simulink model "Vehicle_Dynamics_Tests_org"  (Simulink 10.0)
settings: Solver=ode15s  StartTime=0.0  StopTime=10  MaxStep=0.01  RelTol=1e-4  AbsTol=1e-4  EnableMultiTasking=on
PostLoadFcn:
  | Configure_TNO_Tire_Test('handling');
undefined symbols (not defined in the file): angparking, delta, is, TNO_Veh_PARAM, tparking, tswd, tvxset, vxset, X, Y, Z
libraries: sm_lib x54, nesl_utility x25, Delft_Tyre_sm2glib x16
(part 2 of 2)

== system Vehicle_Dynamics_Tests_org/HubRF ==
  Hub : sm_lib/Body Elements/Cylindrical Solid  GraphicAmbientColor=[0.15 0.15 0.15 1.0]  BasedOnType=Density  CenterOfMass=[0 0 0]  CenterOfMassUnits=m  GraphicDiffuseColor=[0.2 0.8 1.0]  CylinderLength=TNO_Veh_PARAM.Hub.Length  CylinderLengthUnits=m  CylinderRadius=TNO_Veh_PARAM.Hub.Radius  CylinderRadiusUnits=m  Density=1000  DensityUnits=kg/(m^3)  DoExposeReferenceFrame=on  GraphicEmissiveColor=[0.0 0.0 0.0 1.0]  ExportEntireGeometry=off  SerializedFrames=<Frames/>  MarkerShape=Sphere  MarkerSize=10  GraphicType=FromGeometry  InertiaType=CalculateFromGeometry  Mass=1  MassUnits=kg  MomentsOfInertia=[1 1 1]  MomentsOfInertiaUnits=kg*m^2  GraphicOpacity=1.0  ProductsOfInertia=[0 0 0]  ProductsOfInertiaUnits=kg*m^2  GraphicShininess=75  GraphicSpecularColor=[0.5 0.5 0.5 1.0]  GraphicVisPropType=SimpleVisualProperties
  Transform (Whl) : sm_lib/Frames and Transforms/Rigid Transform  TranslationMethod=None  TranslationStandardOffset=0  TranslationLengthUnit=m  TranslationStandardAxis=+Z  TranslationCartesianOffset=[0 0 0]  TranslationROffset=0  TranslationROffsetUnits=m  TranslationZOffset=0  TranslationZOffsetUnits=m  TranslationThetaOffset=0  TranslationThetaOffsetUnits=deg  RotationMethod=StandardAxis  RotationAngleUnits=deg  RotationStandardAxis=-X  RotationAngle=90  RotationArbitraryAxis=[0 0 1]  FollAlignAxisA=+X  BaseAlignAxisA=+Y  FollAlignAxisB=+Y  BaseAlignAxisB=+Z  RotationSequenceAxes=FollowerAxes  RotationSequence=XYX  RotationSequenceAngles=[0 0 0]  RotationSequenceAnglesUnits=deg  RotationMatrix=[1 0 0; 0 1 0; 0 0 1]
  Transform1 (Whl) : sm_lib/Frames and Transforms/Rigid Transform  TranslationMethod=None  TranslationStandardOffset=0  TranslationLengthUnit=m  TranslationStandardAxis=+Z  TranslationCartesianOffset=[0 0 0]  TranslationROffset=0  TranslationROffsetUnits=m  TranslationZOffset=0  TranslationZOffsetUnits=m  TranslationThetaOffset=0  TranslationThetaOffsetUnits=deg  RotationMethod=StandardAxis  RotationAngleUnits=deg  RotationStandardAxis=+Z  RotationAngle=180  RotationArbitraryAxis=[0 0 1]  FollAlignAxisA=+X  BaseAlignAxisA=+Y  FollAlignAxisB=+Y  BaseAlignAxisB=+Z  RotationSequenceAxes=FollowerAxes  RotationSequence=XYX  RotationSequenceAngles=[0 0 0]  RotationSequenceAnglesUnits=deg  RotationMatrix=[1 0 0; 0 1 0; 0 0 1]
  Axle : PMIOPort  Side=Left
  Whl : PMIOPort  Port=2  Side=Right
  connections:
  Hub/RConn1 -- Axle/RConn1 -- Transform1 (Whl)/LConn1
  Transform (Whl)/LConn1 -- Transform1 (Whl)/RConn1
  Whl/RConn1 -- Transform (Whl)/RConn1

== system Vehicle_Dynamics_Tests_org/Maneuver selection ==

== system Vehicle_Dynamics_Tests_org/Plot Tire Results ==

== system Vehicle_Dynamics_Tests_org/RA Housing ==
  Axle Ctr : sm_lib/Body Elements/Cylindrical Solid  GraphicAmbientColor=[0.15 0.15 0.15 1.0]  BasedOnType=Density  CenterOfMass=[0 0 0]  CenterOfMassUnits=m  GraphicDiffuseColor=[0.6 0.6 0.6]  CylinderLength=TNO_Veh_PARAM.Axle_Housing.Length  CylinderLengthUnits=m  CylinderRadius=TNO_Veh_PARAM.Axle_Housing.Radius  CylinderRadiusUnits=m  Density=1000  DensityUnits=kg/(m^3)  DoExposeReferenceFrame=on  GraphicEmissiveColor=[0.0 0.0 0.0 1.0]  ExportEntireGeometry=off  SerializedFrames=<Frames/>  MarkerShape=Sphere  MarkerSize=10  GraphicType=FromGeometry  InertiaType=CalculateFromGeometry  Mass=1  MassUnits=kg  MomentsOfInertia=[1 1 1]  MomentsOfInertiaUnits=kg*m^2  GraphicOpacity=1.0  ProductsOfInertia=[0 0 0]  ProductsOfInertiaUnits=kg*m^2  GraphicShininess=75  GraphicSpecularColor=[0.5 0.5 0.5 1.0]  GraphicVisPropType=SimpleVisualProperties
  Transform (Body) : sm_lib/Frames and Transforms/Rigid Transform  TranslationMethod=None  TranslationStandardOffset=0  TranslationLengthUnit=m  TranslationStandardAxis=+Z  TranslationCartesianOffset=[0 0.05 0]  TranslationROffset=0  TranslationROffsetUnits=m  TranslationZOffset=0  TranslationZOffsetUnits=m  TranslationThetaOffset=0  TranslationThetaOffsetUnits=deg  RotationMethod=StandardAxis  RotationAngleUnits=deg  RotationStandardAxis=+X  RotationAngle=90  RotationArbitraryAxis=[0 0 1]  FollAlignAxisA=+X  BaseAlignAxisA=+Y  FollAlignAxisB=+Y  BaseAlignAxisB=+Z  RotationSequenceAxes=FollowerAxes  RotationSequence=XYX  RotationSequenceAngles=[0 0 0]  RotationSequenceAnglesUnits=deg  RotationMatrix=[1 0 0; 0 1 0; 0 0 1]
  Transform (RA) : sm_lib/Frames and Transforms/Rigid Transform  TranslationMethod=StandardAxis  TranslationStandardOffset=TNO_Veh_PARAM.Suspension.RA.Roll.Height  TranslationLengthUnit=m  TranslationStandardAxis=+Y  TranslationCartesianOffset=[0 0.05 0]  TranslationROffset=0  TranslationROffsetUnits=m  TranslationZOffset=0  TranslationZOffsetUnits=m  TranslationThetaOffset=0  TranslationThetaOffsetUnits=deg  RotationMethod=StandardAxis  RotationAngleUnits=deg  RotationStandardAxis=+Y  RotationAngle=90  RotationArbitraryAxis=[0 0 1]  FollAlignAxisA=+X  BaseAlignAxisA=+Y  FollAlignAxisB=+Y  BaseAlignAxisB=+Z  RotationSequenceAxes=FollowerAxes  RotationSequence=XYX  RotationSequenceAngles=[0 0 0]  RotationSequenceAnglesUnits=deg  RotationMatrix=[1 0 0; 0 1 0; 0 0 1]
  Body : PMIOPort  Side=Left
  RA : PMIOPort  Port=2  Side=Right
  connections:
  RA/RConn1 -- Transform (RA)/RConn1
  Transform (Body)/LConn1 -- Axle Ctr/RConn1 -- Transform (RA)/LConn1
  Transform (Body)/RConn1 -- Body/RConn1

== system Vehicle_Dynamics_Tests_org/RHeave ==
  PS-Simulink Converter14 : nesl_utility/PS-Simulink Converter  PhysicalDomain=network_engine_domain  SubClassName=ps_output  LeftPortType=input  RightPortType=output  PseudoPeriodic=off  Frequencies=[]  Unit=m  AffineConversion=off
  To Workspace4 : ToWorkspace  VariableName=RAheave  SampleTime=-1
  Conn1 : PMIOPort  Side=Left
  wires:
  PS-Simulink Converter14/1 -> To Workspace4/1
  connections:
  Conn1/RConn1 -- PS-Simulink Converter14/LConn1

== system Vehicle_Dynamics_Tests_org/RRoll ==
  PS-Simulink Converter16 : nesl_utility/PS-Simulink Converter  PhysicalDomain=network_engine_domain  SubClassName=ps_output  LeftPortType=input  RightPortType=output  PseudoPeriodic=off  Frequencies=[]  Unit=deg  AffineConversion=off
  To Workspace2 : ToWorkspace  VariableName=RAroll  SampleTime=-1
  Conn1 : PMIOPort  Side=Right
  wires:
  PS-Simulink Converter16/1 -> To Workspace2/1
  connections:
  Conn1/RConn1 -- PS-Simulink Converter16/LConn1

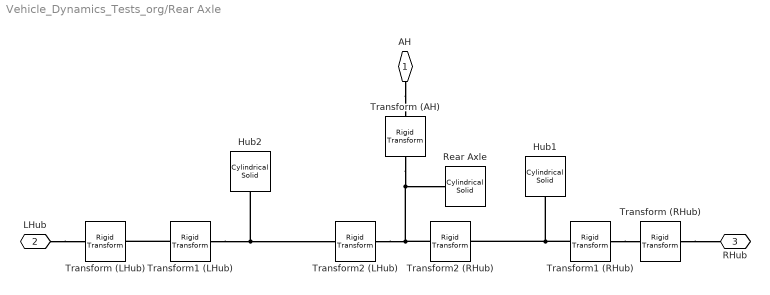
== system Vehicle_Dynamics_Tests_org/Rear Axle ==
  Hub1 : sm_lib/Body Elements/Cylindrical Solid  GraphicAmbientColor=[0.15 0.15 0.15 1.0]  BasedOnType=Density  CenterOfMass=[0 0 0]  CenterOfMassUnits=m  GraphicDiffuseColor=[0.2 0.8 1.0]  CylinderLength=TNO_Veh_PARAM.Hub.Length  CylinderLengthUnits=m  CylinderRadius=TNO_Veh_PARAM.Hub.Radius  CylinderRadiusUnits=m  Density=1000  DensityUnits=kg/(m^3)  DoExposeReferenceFrame=on  GraphicEmissiveColor=[0.0 0.0 0.0 1.0]  ExportEntireGeometry=off  SerializedFrames=<Frames/>  MarkerShape=Sphere  MarkerSize=10  GraphicType=FromGeometry  InertiaType=CalculateFromGeometry  Mass=1  MassUnits=kg  MomentsOfInertia=[1 1 1]  MomentsOfInertiaUnits=kg*m^2  GraphicOpacity=1.0  ProductsOfInertia=[0 0 0]  ProductsOfInertiaUnits=kg*m^2  GraphicShininess=75  GraphicSpecularColor=[0.5 0.5 0.5 1.0]  GraphicVisPropType=SimpleVisualProperties
  Hub2 : sm_lib/Body Elements/Cylindrical Solid  GraphicAmbientColor=[0.15 0.15 0.15 1.0]  BasedOnType=Density  CenterOfMass=[0 0 0]  CenterOfMassUnits=m  GraphicDiffuseColor=[0.2 0.8 1.0]  CylinderLength=TNO_Veh_PARAM.Hub.Length  CylinderLengthUnits=m  CylinderRadius=TNO_Veh_PARAM.Hub.Radius  CylinderRadiusUnits=m  Density=1000  DensityUnits=kg/(m^3)  DoExposeReferenceFrame=on  GraphicEmissiveColor=[0.0 0.0 0.0 1.0]  ExportEntireGeometry=off  SerializedFrames=<Frames/>  MarkerShape=Sphere  MarkerSize=10  GraphicType=FromGeometry  InertiaType=CalculateFromGeometry  Mass=1  MassUnits=kg  MomentsOfInertia=[1 1 1]  MomentsOfInertiaUnits=kg*m^2  GraphicOpacity=1.0  ProductsOfInertia=[0 0 0]  ProductsOfInertiaUnits=kg*m^2  GraphicShininess=75  GraphicSpecularColor=[0.5 0.5 0.5 1.0]  GraphicVisPropType=SimpleVisualProperties
  Rear Axle : sm_lib/Body Elements/Cylindrical Solid  GraphicAmbientColor=[0.15 0.15 0.15 1.0]  BasedOnType=Density  CenterOfMass=[0 0 0]  CenterOfMassUnits=m  GraphicDiffuseColor=[0.6 0.6 0.6]  CylinderLength=TNO_Veh_PARAM.Axle.RA.Length  CylinderLengthUnits=m  CylinderRadius=TNO_Veh_PARAM.Axle.RA.Radius  CylinderRadiusUnits=m  Density=1000  DensityUnits=kg/(m^3)  DoExposeReferenceFrame=on  GraphicEmissiveColor=[0.0 0.0 0.0 1.0]  ExportEntireGeometry=off  SerializedFrames=<Frames/>  MarkerShape=Sphere  MarkerSize=10  GraphicType=FromGeometry  InertiaType=Custom  Mass=TNO_Veh_PARAM.Axle.RA.Mass  MassUnits=kg  MomentsOfInertia=TNO_Veh_PARAM.Axle.RA.Inertia  MomentsOfInertiaUnits=kg*m^2  GraphicOpacity=1.0  ProductsOfInertia=[0 0 0]  ProductsOfInertiaUnits=kg*m^2  GraphicShininess=75  GraphicSpecularColor=[0.5 0.5 0.5 1.0]  GraphicVisPropType=SimpleVisualProperties
  Transform (AH) : sm_lib/Frames and Transforms/Rigid Transform  TranslationMethod=StandardAxis  TranslationStandardOffset=TNO_Veh_PARAM.Axle.RA.Height  TranslationLengthUnit=m  TranslationStandardAxis=+Y  TranslationCartesianOffset=[0 0.225 0]  TranslationROffset=0  TranslationROffsetUnits=m  TranslationZOffset=0  TranslationZOffsetUnits=m  TranslationThetaOffset=0  TranslationThetaOffsetUnits=deg  RotationMethod=StandardAxis  RotationAngleUnits=deg  RotationStandardAxis=+Y  RotationAngle=-90  RotationArbitraryAxis=[0 0 1]  FollAlignAxisA=+X  BaseAlignAxisA=+Y  FollAlignAxisB=+Y  BaseAlignAxisB=+Z  RotationSequenceAxes=FollowerAxes  RotationSequence=XYX  RotationSequenceAngles=[0 0 0]  RotationSequenceAnglesUnits=deg  RotationMatrix=[1 0 0; 0 1 0; 0 0 1]
  Transform (LHub) : sm_lib/Frames and Transforms/Rigid Transform  TranslationMethod=None  TranslationStandardOffset=0  TranslationLengthUnit=m  TranslationStandardAxis=+Z  TranslationCartesianOffset=[0 0 0]  TranslationROffset=0  TranslationROffsetUnits=m  TranslationZOffset=0  TranslationZOffsetUnits=m  TranslationThetaOffset=0  TranslationThetaOffsetUnits=deg  RotationMethod=StandardAxis  RotationAngleUnits=deg  RotationStandardAxis=-X  RotationAngle=90  RotationArbitraryAxis=[0 0 1]  FollAlignAxisA=+X  BaseAlignAxisA=+Y  FollAlignAxisB=+Y  BaseAlignAxisB=+Z  RotationSequenceAxes=FollowerAxes  RotationSequence=XYX  RotationSequenceAngles=[0 0 0]  RotationSequenceAnglesUnits=deg  RotationMatrix=[1 0 0; 0 1 0; 0 0 1]
  Transform (RHub) : sm_lib/Frames and Transforms/Rigid Transform  TranslationMethod=None  TranslationStandardOffset=0  TranslationLengthUnit=m  TranslationStandardAxis=+Z  TranslationCartesianOffset=[0 0 0]  TranslationROffset=0  TranslationROffsetUnits=m  TranslationZOffset=0  TranslationZOffsetUnits=m  TranslationThetaOffset=0  TranslationThetaOffsetUnits=deg  RotationMethod=StandardAxis  RotationAngleUnits=deg  RotationStandardAxis=-X  RotationAngle=90  RotationArbitraryAxis=[0 0 1]  FollAlignAxisA=+X  BaseAlignAxisA=+Y  FollAlignAxisB=+Y  BaseAlignAxisB=+Z  RotationSequenceAxes=FollowerAxes  RotationSequence=XYX  RotationSequenceAngles=[0 0 0]  RotationSequenceAnglesUnits=deg  RotationMatrix=[1 0 0; 0 1 0; 0 0 1]
  Transform1 (LHub) : sm_lib/Frames and Transforms/Rigid Transform  TranslationMethod=None  TranslationStandardOffset=0  TranslationLengthUnit=m  TranslationStandardAxis=+Z  TranslationCartesianOffset=[0 0 0]  TranslationROffset=0  TranslationROffsetUnits=m  TranslationZOffset=0  TranslationZOffsetUnits=m  TranslationThetaOffset=0  TranslationThetaOffsetUnits=deg  RotationMethod=StandardAxis  RotationAngleUnits=deg  RotationStandardAxis=+Z  RotationAngle=180  RotationArbitraryAxis=[0 0 1]  FollAlignAxisA=+X  BaseAlignAxisA=+Y  FollAlignAxisB=+Y  BaseAlignAxisB=+Z  RotationSequenceAxes=FollowerAxes  RotationSequence=XYX  RotationSequenceAngles=[0 0 0]  RotationSequenceAnglesUnits=deg  RotationMatrix=[1 0 0; 0 1 0; 0 0 1]
  Transform1 (RHub) : sm_lib/Frames and Transforms/Rigid Transform  TranslationMethod=None  TranslationStandardOffset=0  TranslationLengthUnit=m  TranslationStandardAxis=+Z  TranslationCartesianOffset=[0 0 0]  TranslationROffset=0  TranslationROffsetUnits=m  TranslationZOffset=0  TranslationZOffsetUnits=m  TranslationThetaOffset=0  TranslationThetaOffsetUnits=deg  RotationMethod=StandardAxis  RotationAngleUnits=deg  RotationStandardAxis=+Z  RotationAngle=180  RotationArbitraryAxis=[0 0 1]  FollAlignAxisA=+X  BaseAlignAxisA=+Y  FollAlignAxisB=+Y  BaseAlignAxisB=+Z  RotationSequenceAxes=FollowerAxes  RotationSequence=XYX  RotationSequenceAngles=[0 0 0]  RotationSequenceAnglesUnits=deg  RotationMatrix=[1 0 0; 0 1 0; 0 0 1]
  Transform2 (LHub) : sm_lib/Frames and Transforms/Rigid Transform  TranslationMethod=StandardAxis  TranslationStandardOffset=-TNO_Veh_PARAM.WheelBase/2  TranslationLengthUnit=m  TranslationStandardAxis=+Z  TranslationCartesianOffset=[0 0 0]  TranslationROffset=0  TranslationROffsetUnits=m  TranslationZOffset=0  TranslationZOffsetUnits=m  TranslationThetaOffset=0  TranslationThetaOffsetUnits=deg  RotationMethod=StandardAxis  RotationAngleUnits=deg  RotationStandardAxis=+X  RotationAngle=90  RotationArbitraryAxis=[0 0 1]  FollAlignAxisA=+X  BaseAlignAxisA=+Y  FollAlignAxisB=+Y  BaseAlignAxisB=+Z  RotationSequenceAxes=FollowerAxes  RotationSequence=XYX  RotationSequenceAngles=[0 0 0]  RotationSequenceAnglesUnits=deg  RotationMatrix=[1 0 0; 0 1 0; 0 0 1]
  Transform2 (RHub) : sm_lib/Frames and Transforms/Rigid Transform  TranslationMethod=StandardAxis  TranslationStandardOffset=TNO_Veh_PARAM.WheelBase/2  TranslationLengthUnit=m  TranslationStandardAxis=+Z  TranslationCartesianOffset=[0 0 0]  TranslationROffset=0  TranslationROffsetUnits=m  TranslationZOffset=0  TranslationZOffsetUnits=m  TranslationThetaOffset=0  TranslationThetaOffsetUnits=deg  RotationMethod=StandardAxis  RotationAngleUnits=deg  RotationStandardAxis=+X  RotationAngle=90  RotationArbitraryAxis=[0 0 1]  FollAlignAxisA=+X  BaseAlignAxisA=+Y  FollAlignAxisB=+Y  BaseAlignAxisB=+Z  RotationSequenceAxes=FollowerAxes  RotationSequence=XYX  RotationSequenceAngles=[0 0 0]  RotationSequenceAnglesUnits=deg  RotationMatrix=[1 0 0; 0 1 0; 0 0 1]
  AH : PMIOPort  Side=Left
  LHub : PMIOPort  Port=2  Side=Right
  RHub : PMIOPort  Port=3  Side=Right
  connections:
  AH/RConn1 -- Transform (AH)/RConn1
  Transform2 (LHub)/LConn1 -- Transform (AH)/LConn1 -- Rear Axle/RConn1 -- Transform2 (RHub)/LConn1
  Transform1 (RHub)/LConn1 -- Transform2 (RHub)/RConn1 -- Hub1/RConn1
  Transform1 (LHub)/LConn1 -- Transform2 (LHub)/RConn1 -- Hub2/RConn1
  Transform1 (RHub)/RConn1 -- Transform (RHub)/LConn1
  Transform (RHub)/RConn1 -- RHub/RConn1
  Transform1 (LHub)/RConn1 -- Transform (LHub)/LConn1
  LHub/RConn1 -- Transform (LHub)/RConn1

== system Vehicle_Dynamics_Tests_org/Sensing ==
  Mux : Mux
  Fz : Outport
  wires:
  [RR_Fz] -> Mux/4
  Mux/1 -> Fz/1
  [LF_Fz] -> Mux/1
  [RF_Fz] -> Mux/2
  [LR_Fz] -> Mux/3

== system Vehicle_Dynamics_Tests_org/Steering Input ==
  note: 1) Only subsystems can be added as variant choices at this level
      | 2) Blocks cannot be connected at this level as connectivity is
      | automatically determined at simulation, based on the active variant
  No Steer : Subsystem  VariantControl=NoSteer
  Parking : Subsystem  VariantControl=Parking
  Sine With Dwell : Subsystem  VariantControl=SineWithDwell
  Slalom : Subsystem  VariantControl=Slalom
  Step Steer : Subsystem  VariantControl=StepSteer
  L : PMIOPort  Side=Right
  R : PMIOPort  Port=2  Side=Right

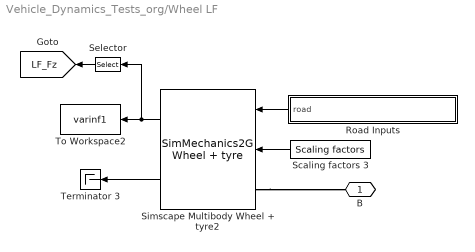
== system Vehicle_Dynamics_Tests_org/Wheel LF ==
  Road Inputs : Subsystem  VariantControlMode=Label  Variant=on  LabelModeActiveChoice=NonMoving
  Scaling factors 3 : Delft_Tyre_sm2glib/SimMechanics 2G/Scaling factors  LMUX=1  LKX=1  LMUY=1  LKY=1  LKYC=1  LTR=1  LKZC=1
  Selector : Selector  InputPortWidth=40  IndexOptions=Index vector (dialog)  Indices=[3]  OutputSizes=1
  Simscape Multibody Wheel + tyre2 : Delft_Tyre_sm2glib/SimMechanics 2G/SimMechanics2G Wheel + tyre  Tag=SimMechanics Wheel + tyre  idtyre=1  inertia=[10 1 2]  tpfname=which('TNO_car205_60R15.tir')  rdfname=which('TNO_FlatRoad.rdf')  side_mode=(1xxx) left  cnt_mode=(x1xx) smooth road  dyn_mode=(xx2x) relaxation behaviour - non-linear  mf_mode=(xxx4) combined  use_mode=1e8  disp_debug=off
  Terminator 3 : Terminator
  To Workspace2 : ToWorkspace  VariableName=varinf1  SampleTime=-1
  B : PMIOPort  Side=Right
  tag scope: LF_Fz=global
  wires:
  Scaling factors 3/1 -> Simscape Multibody Wheel + tyre2/2
  Road Inputs/1(road) -> Simscape Multibody Wheel + tyre2/1
  Simscape Multibody Wheel + tyre2/1 -> Selector/1, To Workspace2/1
  Simscape Multibody Wheel + tyre2/2 -> Terminator 3/1
  Selector/1 -> [LF_Fz]
  connections:
  Simscape Multibody Wheel + tyre2/LConn1 -- B/RConn1

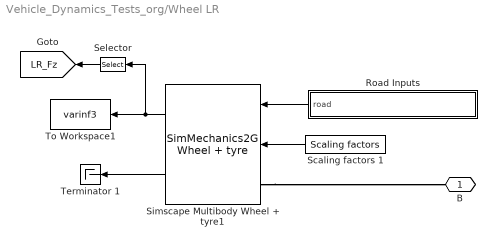
== system Vehicle_Dynamics_Tests_org/Wheel LR ==
  Road Inputs : Subsystem  VariantControlMode=Label  Variant=on  LabelModeActiveChoice=NonMoving
  Scaling factors 1 : Delft_Tyre_sm2glib/SimMechanics 2G/Scaling factors  LMUX=1  LKX=1  LMUY=1  LKY=1  LKYC=1  LTR=1  LKZC=1
  Selector : Selector  InputPortWidth=40  IndexOptions=Index vector (dialog)  Indices=[3]  OutputSizes=1
  Simscape Multibody Wheel + tyre1 : Delft_Tyre_sm2glib/SimMechanics 2G/SimMechanics2G Wheel + tyre  Tag=SimMechanics Wheel + tyre  idtyre=3  inertia=[10 1 2]  tpfname=which('TNO_car205_60R15.tir')  rdfname=which('TNO_FlatRoad.rdf')  side_mode=(1xxx) left  cnt_mode=(x1xx) smooth road  dyn_mode=(xx2x) relaxation behaviour - non-linear  mf_mode=(xxx4) combined  use_mode=1e8  disp_debug=off
  Terminator 1 : Terminator
  To Workspace1 : ToWorkspace  VariableName=varinf3  SampleTime=-1
  B : PMIOPort  Side=Right
  tag scope: LR_Fz=global
  wires:
  Scaling factors 1/1 -> Simscape Multibody Wheel + tyre1/2
  Road Inputs/1(road) -> Simscape Multibody Wheel + tyre1/1
  Simscape Multibody Wheel + tyre1/1 -> Selector/1, To Workspace1/1
  Simscape Multibody Wheel + tyre1/2 -> Terminator 1/1
  Selector/1 -> [LR_Fz]
  connections:
  Simscape Multibody Wheel + tyre1/LConn1 -- B/RConn1

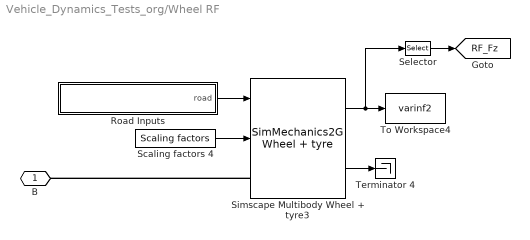
== system Vehicle_Dynamics_Tests_org/Wheel RF ==
  Road Inputs : Subsystem  VariantControlMode=Label  Variant=on  LabelModeActiveChoice=NonMoving
  Scaling factors 4 : Delft_Tyre_sm2glib/SimMechanics 2G/Scaling factors  LMUX=1  LKX=1  LMUY=1  LKY=1  LKYC=1  LTR=1  LKZC=1
  Selector : Selector  InputPortWidth=40  IndexOptions=Index vector (dialog)  Indices=[3]  OutputSizes=1
  Simscape Multibody Wheel + tyre3 : Delft_Tyre_sm2glib/SimMechanics 2G/SimMechanics2G Wheel + tyre  Tag=SimMechanics Wheel + tyre  idtyre=2  inertia=[10 1 2]  tpfname=which('TNO_car205_60R15.tir')  rdfname=which('TNO_FlatRoad.rdf')  side_mode=(2xxx) right  cnt_mode=(x1xx) smooth road  dyn_mode=(xx2x) relaxation behaviour - non-linear  mf_mode=(xxx4) combined  use_mode=1e8  disp_debug=off
  Terminator 4 : Terminator
  To Workspace4 : ToWorkspace  VariableName=varinf2  SampleTime=-1
  B : PMIOPort  Side=Left
  tag scope: RF_Fz=global
  wires:
  Scaling factors 4/1 -> Simscape Multibody Wheel + tyre3/2
  Road Inputs/1(road) -> Simscape Multibody Wheel + tyre3/1
  Simscape Multibody Wheel + tyre3/1 -> Selector/1, To Workspace4/1
  Simscape Multibody Wheel + tyre3/2 -> Terminator 4/1
  Selector/1 -> [RF_Fz]
  connections:
  Simscape Multibody Wheel + tyre3/LConn1 -- B/RConn1

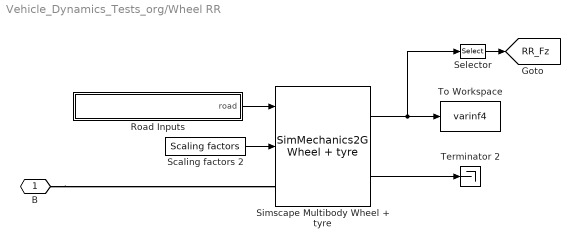
== system Vehicle_Dynamics_Tests_org/Wheel RR ==
  Road Inputs : Subsystem  VariantControlMode=Label  Variant=on  LabelModeActiveChoice=NonMoving
  Scaling factors 2 : Delft_Tyre_sm2glib/SimMechanics 2G/Scaling factors  LMUX=1  LKX=1  LMUY=1  LKY=1  LKYC=1  LTR=1  LKZC=1
  Selector : Selector  InputPortWidth=40  IndexOptions=Index vector (dialog)  Indices=[3]  OutputSizes=1
  Simscape Multibody Wheel + tyre : Delft_Tyre_sm2glib/SimMechanics 2G/SimMechanics2G Wheel + tyre  Tag=SimMechanics Wheel + tyre  idtyre=4  inertia=[10 1 2]  tpfname=which('TNO_car205_60R15.tir')  rdfname=which('TNO_FlatRoad.rdf')  side_mode=(2xxx) right  cnt_mode=(x1xx) smooth road  dyn_mode=(xx2x) relaxation behaviour - non-linear  mf_mode=(xxx4) combined  use_mode=1e8  disp_debug=off
  Terminator 2 : Terminator
  To Workspace : ToWorkspace  VariableName=varinf4  SampleTime=-1
  B : PMIOPort  Side=Left
  tag scope: RR_Fz=global
  wires:
  Scaling factors 2/1 -> Simscape Multibody Wheel + tyre/2
  Road Inputs/1(road) -> Simscape Multibody Wheel + tyre/1
  Simscape Multibody Wheel + tyre/2 -> Terminator 2/1
  Simscape Multibody Wheel + tyre/1 -> Selector/1, To Workspace/1
  Selector/1 -> [RR_Fz]
  connections:
  B/RConn1 -- Simscape Multibody Wheel + tyre/LConn1

== system Vehicle_Dynamics_Tests_org/World ==
  Mechanism Configuration : sm_lib/Utilities/Mechanism Configuration  UniformGravity=Constant  GravityVector=[0 0 -10]  GravityUnits=m/s^2  LinearizationDelta=0.001
  Road : Subsystem  VariantControlMode=Label  Variant=on  LabelModeActiveChoice=NoRoad
  Solver Configuration : nesl_utility/Solver Configuration  PhysicalDomain=network_engine_domain  SubClassName=solver  LeftPortType=input  RightPortType=generic  Tones=[]  Harmonics=[]  SimulateNoise=off  Profile=off  UseLocalSampling=off  EnableSwitchedLinearOptims=on  FrequencyDomain=off  UseCCode=off  RelTol=0.001  AbsTol=1e-06  MinStep=1e-09  ToWorkspace=off  RevertToSquareIcSolve=off  NumHomotopyIterations=100  PhasorMode=off  PhasorModeNumHarmonics=1  DoDC=off  ResidualTolerance=1e-9  UseLocalSolver=off  LocalSolverChoice=NE_BACKWARD_EULER_ADVANCER  LocalSolverSampleTime=.001  DoFixedCost=off  MaxNonlinIter=3  MaxModeIter=2  LinearAlgebra=Sparse  EquationFormulation=NE_TIME_EF  DelaysMemoryBudget=1024  AutomaticFiltering=on  FilteringTimeConstant=0.001  PartitionStorageMethod=AS_NEEDED  PartitionMemoryBudget=1024  PartitionMethod=FAST
  Transform (F) : sm_lib/Frames and Transforms/Rigid Transform  TranslationMethod=Cartesian  TranslationStandardOffset=0.55  TranslationLengthUnit=m  TranslationStandardAxis=+Z  TranslationCartesianOffset=[-TNO_Veh_PARAM.Body.Length/2 0 TNO_Veh_PARAM.Body.Height]  TranslationROffset=0  TranslationROffsetUnits=m  TranslationZOffset=0  TranslationZOffsetUnits=m  TranslationThetaOffset=0  TranslationThetaOffsetUnits=deg  RotationMethod=None  RotationAngleUnits=deg  RotationStandardAxis=+Y  RotationAngle=0  RotationArbitraryAxis=[0 0 1]  FollAlignAxisA=+X  BaseAlignAxisA=+Y  FollAlignAxisB=+Y  BaseAlignAxisB=+Z  RotationSequenceAxes=FollowerAxes  RotationSequence=XYX  RotationSequenceAngles=[0 0 0]  RotationSequenceAnglesUnits=deg  RotationMatrix=[1 0 0; 0 1 0; 0 0 1]
  World Frame : sm_lib/Frames and Transforms/World Frame
  F : PMIOPort  Side=Left
  connections:
  Transform (F)/RConn1 -- F/RConn1
  World Frame/RConn1 -- Road/RConn1 -- Transform (F)/LConn1 -- Solver Configuration/RConn1 -- Mechanism Configuration/RConn1

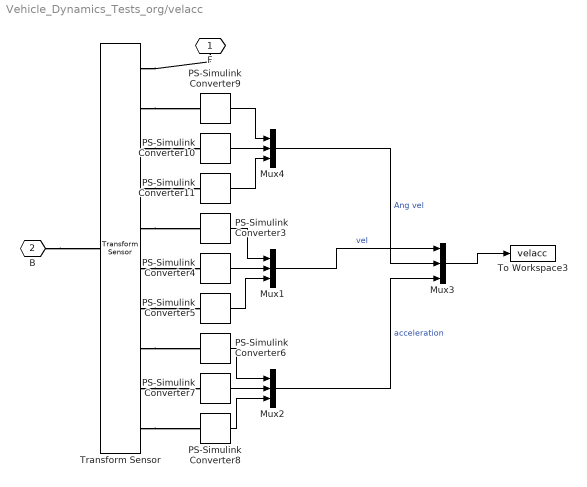
== system Vehicle_Dynamics_Tests_org/velacc ==
  Mux{1..4} (4 alike) : Mux  Inputs=3
  PS-Simulink Converter10 : nesl_utility/PS-Simulink Converter  PhysicalDomain=network_engine_domain  SubClassName=ps_output  LeftPortType=input  RightPortType=output  PseudoPeriodic=off  Frequencies=[]  Unit=deg/s  AffineConversion=off
  PS-Simulink Converter11 : nesl_utility/PS-Simulink Converter  PhysicalDomain=network_engine_domain  SubClassName=ps_output  LeftPortType=input  RightPortType=output  PseudoPeriodic=off  Frequencies=[]  Unit=deg/s  AffineConversion=off
  PS-Simulink Converter3 : nesl_utility/PS-Simulink Converter  PhysicalDomain=network_engine_domain  SubClassName=ps_output  LeftPortType=input  RightPortType=output  PseudoPeriodic=off  Frequencies=[]  Unit=m/s  AffineConversion=off
  PS-Simulink Converter4 : nesl_utility/PS-Simulink Converter  PhysicalDomain=network_engine_domain  SubClassName=ps_output  LeftPortType=input  RightPortType=output  PseudoPeriodic=off  Frequencies=[]  Unit=m/s  AffineConversion=off
  PS-Simulink Converter5 : nesl_utility/PS-Simulink Converter  PhysicalDomain=network_engine_domain  SubClassName=ps_output  LeftPortType=input  RightPortType=output  PseudoPeriodic=off  Frequencies=[]  Unit=m/s  AffineConversion=off
  PS-Simulink Converter6 : nesl_utility/PS-Simulink Converter  PhysicalDomain=network_engine_domain  SubClassName=ps_output  LeftPortType=input  RightPortType=output  PseudoPeriodic=off  Frequencies=[]  Unit=m/s^2  AffineConversion=off
  PS-Simulink Converter7 : nesl_utility/PS-Simulink Converter  PhysicalDomain=network_engine_domain  SubClassName=ps_output  LeftPortType=input  RightPortType=output  PseudoPeriodic=off  Frequencies=[]  Unit=m/s^2  AffineConversion=off
  PS-Simulink Converter8 : nesl_utility/PS-Simulink Converter  PhysicalDomain=network_engine_domain  SubClassName=ps_output  LeftPortType=input  RightPortType=output  PseudoPeriodic=off  Frequencies=[]  Unit=m/s^2  AffineConversion=off
  PS-Simulink Converter9 : nesl_utility/PS-Simulink Converter  PhysicalDomain=network_engine_domain  SubClassName=ps_output  LeftPortType=input  RightPortType=output  PseudoPeriodic=off  Frequencies=[]  Unit=deg/s  AffineConversion=off
  To Workspace3 : ToWorkspace  VariableName=velacc  SampleTime=-1
  Transform Sensor : sm_lib/Frames and Transforms/Transform Sensor  MeasurementFrame=NonRotatingFollower  SenseAngle=off  SenseAxis=off  SenseAngle1=off  SenseAngle2=off  SenseAngle3=off  SenseQ=off  SenseR=off  SenseOmegaX=on  SenseOmegaY=on  SenseOmegaZ=on  SenseOmega1=off  SenseOmega2=off  SenseOmega3=off  SenseQDot=off  SenseRDot=off  SenseAlphaX=off  SenseAlphaY=off  SenseAlphaZ=off  SenseAlpha1=off  SenseAlpha2=off  SenseAlpha3=off  SenseQDDot=off  SenseRDDot=off  SenseX=off  SenseY=off  SenseZ=off  SenseRad=off  SenseAzim=off  SenseDist=off  SenseInc=off  SenseXDot=on  SenseYDot=on  SenseZDot=on  SenseRadDot=off  SenseAzimDot=off  SenseDistDot=off  SenseIncDot=off  SenseXDDot=on  SenseYDDot=on  SenseZDDot=on  SenseRadDDot=off  SenseAzimDDot=off  SenseDistDDot=off  SenseIncDDot=off
  F : PMIOPort  Side=Right
  B : PMIOPort  Port=2  Side=Left
  wires:
  PS-Simulink Converter5/1 -> Mux1/3
  PS-Simulink Converter6/1 -> Mux2/1
  Mux4/1 -> Mux3/2  "Ang vel"
  Mux1/1 -> Mux3/1  "vel"
  Mux2/1 -> Mux3/3  "acceleration"
  Mux3/1 -> To Workspace3/1
  PS-Simulink Converter7/1 -> Mux2/2
  PS-Simulink Converter4/1 -> Mux1/2
  PS-Simulink Converter3/1 -> Mux1/1
  PS-Simulink Converter8/1 -> Mux2/3
  PS-Simulink Converter11/1 -> Mux4/3
  PS-Simulink Converter9/1 -> Mux4/1
  PS-Simulink Converter10/1 -> Mux4/2
  connections:
  Transform Sensor/RConn9 -- PS-Simulink Converter7/LConn1
  Transform Sensor/RConn8 -- PS-Simulink Converter6/LConn1
  Transform Sensor/RConn5 -- PS-Simulink Converter3/LConn1
  Transform Sensor/RConn7 -- PS-Simulink Converter5/LConn1
  Transform Sensor/RConn6 -- PS-Simulink Converter4/LConn1
  Transform Sensor/RConn10 -- PS-Simulink Converter8/LConn1
  B/RConn1 -- Transform Sensor/LConn1
  Transform Sensor/RConn1 -- F/RConn1
  Transform Sensor/RConn2 -- PS-Simulink Converter9/LConn1
  Transform Sensor/RConn3 -- PS-Simulink Converter10/LConn1
  Transform Sensor/RConn4 -- PS-Simulink Converter11/LConn1

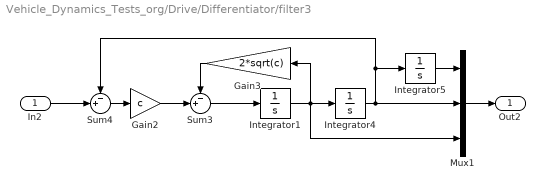
== system Vehicle_Dynamics_Tests_org/Drive/Differentiator/filter3 ==
  In2 : Inport
  Gain2 : Gain  Gain=c  SaturateOnIntegerOverflow=on  OutDataTypeStr=Inherit: Same as input  ParamDataTypeStr=Inherit: Same as input
  Gain3 : Gain  Gain=2*sqrt(c)  SaturateOnIntegerOverflow=on  OutDataTypeStr=Inherit: Same as input  ParamDataTypeStr=Inherit: Same as input
  Integrator1 : Integrator
  Integrator4 : Integrator
  Integrator5 : Integrator  InitialCondition=-1.5
  Mux1 : Mux  Inputs=3
  Sum3 : Sum  Inputs=-+|  SaturateOnIntegerOverflow=on
  Sum4 : Sum  Inputs=-+|  SaturateOnIntegerOverflow=on
  Out2 : Outport
  wires:
  Integrator5/1 -> Mux1/1
  Gain2/1 -> Sum3/2
  Gain3/1 -> Sum3/1
  In2/1 -> Sum4/2
  Sum4/1 -> Gain2/1
  Sum3/1 -> Integrator1/1
  Mux1/1 -> Out2/1
  Integrator4/1 -> Integrator5/1, Sum4/1, Mux1/2
  Integrator1/1 -> Mux1/3, Integrator4/1, Gain3/1

== system Vehicle_Dynamics_Tests_org/Steering Input/No Steer ==
  Constant : Constant  Value=0
  Constant1 : Constant  Value=0
  Simulink-PS Converter : nesl_utility/Simulink-PS Converter  PhysicalDomain=network_engine_domain  SubClassName=ps_input  LeftPortType=input  RightPortType=output  PseudoPeriodic=off  Frequencies=[]  NoiseDistribution=none  NoiseParameters=[]  Unit=rad  AffineConversion=off  FilteringAndDerivatives=filter  SimscapeFilterOrder=2  InputFilterTimeConstant=0.0055  UdotUserProvided=2
  Simulink-PS Converter1 : nesl_utility/Simulink-PS Converter  PhysicalDomain=network_engine_domain  SubClassName=ps_input  LeftPortType=input  RightPortType=output  PseudoPeriodic=off  Frequencies=[]  NoiseDistribution=none  NoiseParameters=[]  Unit=rad  AffineConversion=off  FilteringAndDerivatives=filter  SimscapeFilterOrder=2  InputFilterTimeConstant=0.0055  UdotUserProvided=2
  L : PMIOPort  Side=Right
  R : PMIOPort  Port=2  Side=Right
  wires:
  Constant1/1 -> Simulink-PS Converter/1
  Constant/1 -> Simulink-PS Converter1/1
  connections:
  Simulink-PS Converter1/RConn1 -- L/RConn1
  Simulink-PS Converter/RConn1 -- R/RConn1

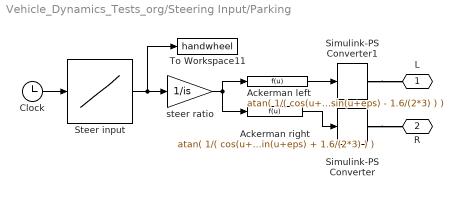
== system Vehicle_Dynamics_Tests_org/Steering Input/Parking ==
  Ackerman left : Fcn  Expr=atan( 1/( cos(u+eps)/sin(u+eps) - 1.6/(2*3) ) )
  Ackerman right : Fcn  Expr=atan( 1/( cos(u+eps)/sin(u+eps) + 1.6/(2*3) ) )
  Clock : Clock
  Simulink-PS Converter : nesl_utility/Simulink-PS Converter  PhysicalDomain=network_engine_domain  SubClassName=ps_input  LeftPortType=input  RightPortType=output  PseudoPeriodic=off  Frequencies=[]  NoiseDistribution=none  NoiseParameters=[]  Unit=rad  AffineConversion=off  FilteringAndDerivatives=filter  SimscapeFilterOrder=2  InputFilterTimeConstant=0.0055  UdotUserProvided=2
  Simulink-PS Converter1 : nesl_utility/Simulink-PS Converter  PhysicalDomain=network_engine_domain  SubClassName=ps_input  LeftPortType=input  RightPortType=output  PseudoPeriodic=off  Frequencies=[]  NoiseDistribution=none  NoiseParameters=[]  Unit=rad  AffineConversion=off  FilteringAndDerivatives=filter  SimscapeFilterOrder=2  InputFilterTimeConstant=0.0055  UdotUserProvided=2
  Steer input : Lookup  InputValues=tparking  Table=angparking
  To Workspace11 : ToWorkspace  VariableName=handwheel  SampleTime=-1
  steer ratio : Gain  Gain=1/is
  L : PMIOPort  Side=Right
  R : PMIOPort  Port=2  Side=Right
  wires:
  Clock/1 -> Steer input/1
  Steer input/1 -> steer ratio/1, To Workspace11/1
  steer ratio/1 -> Ackerman left/1, Ackerman right/1
  Ackerman left/1 -> Simulink-PS Converter1/1
  Ackerman right/1 -> Simulink-PS Converter/1
  connections:
  Simulink-PS Converter/RConn1 -- R/RConn1
  Simulink-PS Converter1/RConn1 -- L/RConn1

== system Vehicle_Dynamics_Tests_org/Steering Input/Sine With Dwell ==
  Clock : Clock
  Simulink-PS Converter : nesl_utility/Simulink-PS Converter  PhysicalDomain=network_engine_domain  SubClassName=ps_input  LeftPortType=input  RightPortType=output  PseudoPeriodic=off  Frequencies=[]  NoiseDistribution=none  NoiseParameters=[]  Unit=rad  AffineConversion=off  FilteringAndDerivatives=filter  SimscapeFilterOrder=2  InputFilterTimeConstant=0.0055  UdotUserProvided=2
  Sine with Dwell Steer input : Lookup  InputValues=tswd  Table=delta
  To Workspace12 : ToWorkspace  VariableName=handwheel  SampleTime=-1
  steer ratio : Gain  Gain=1/is
  L : PMIOPort  Side=Right
  R : PMIOPort  Port=2  Side=Right
  wires:
  Clock/1 -> Sine with Dwell Steer input/1
  Sine with Dwell Steer input/1 -> To Workspace12/1, steer ratio/1
  steer ratio/1 -> Simulink-PS Converter/1
  connections:
  Simulink-PS Converter/RConn1 -- R/RConn1 -- L/RConn1

== system Vehicle_Dynamics_Tests_org/Steering Input/Slalom ==
  Simulink-PS Converter : nesl_utility/Simulink-PS Converter  PhysicalDomain=network_engine_domain  SubClassName=ps_input  LeftPortType=input  RightPortType=output  PseudoPeriodic=off  Frequencies=[]  NoiseDistribution=none  NoiseParameters=[]  Unit=rad  AffineConversion=off  FilteringAndDerivatives=filter  SimscapeFilterOrder=2  InputFilterTimeConstant=0.0055  UdotUserProvided=2
  Sine Wave : Sin  Amplitude=15*(pi/180)  Frequency=4*pi/10  Phase=pi/2+0.03  SampleTime=0
  To Workspace12 : ToWorkspace  VariableName=handwheel  SampleTime=-1
  steer ratio : Gain  Gain=1/is
  L : PMIOPort  Side=Right
  R : PMIOPort  Port=2  Side=Right
  wires:
  steer ratio/1 -> Simulink-PS Converter/1
  Sine Wave/1 -> steer ratio/1, To Workspace12/1
  connections:
  L/RConn1 -- R/RConn1 -- Simulink-PS Converter/RConn1

== system Vehicle_Dynamics_Tests_org/Steering Input/Step Steer ==
  Simulink-PS Converter : nesl_utility/Simulink-PS Converter  PhysicalDomain=network_engine_domain  SubClassName=ps_input  LeftPortType=input  RightPortType=output  PseudoPeriodic=off  Frequencies=[]  NoiseDistribution=none  NoiseParameters=[]  Unit=rad  AffineConversion=off  FilteringAndDerivatives=filter  SimscapeFilterOrder=2  InputFilterTimeConstant=0.0055  UdotUserProvided=2
  Step Steer input : Step  Time=3  After=10*pi/180  SampleTime=0
  L : PMIOPort  Side=Right
  R : PMIOPort  Port=2  Side=Right
  wires:
  Step Steer input/1 -> Simulink-PS Converter/1
  connections:
  Simulink-PS Converter/RConn1 -- R/RConn1 -- L/RConn1

== system Vehicle_Dynamics_Tests_org/Wheel LF/Road Inputs ==
  note: 1) Only subsystems can be added as variant choices at this level
      | 2) Blocks cannot be connected at this level as connectivity is
      | automatically determined at simulation, based on the active variant
  Non-moving road : Delft_Tyre_sm2glib/SimMechanics 2G/Non-moving road  VariantControl=NonMoving  dummy=off
  Test Rig Post : Subsystem  VariantControl=TestRigPost
  road : Outport

== system Vehicle_Dynamics_Tests_org/Wheel LR/Road Inputs ==
  note: 1) Only subsystems can be added as variant choices at this level
      | 2) Blocks cannot be connected at this level as connectivity is
      | automatically determined at simulation, based on the active variant
  Non-moving road : Delft_Tyre_sm2glib/SimMechanics 2G/Non-moving road  VariantControl=NonMoving  dummy=off
  Test Rig Post : Subsystem  VariantControl=TestRigPost
  road : Outport

== system Vehicle_Dynamics_Tests_org/Wheel RF/Road Inputs ==
  note: 1) Only subsystems can be added as variant choices at this level
      | 2) Blocks cannot be connected at this level as connectivity is
      | automatically determined at simulation, based on the active variant
  Non-moving road : Delft_Tyre_sm2glib/SimMechanics 2G/Non-moving road  VariantControl=NonMoving  dummy=off
  Test Rig Post : Subsystem  VariantControl=TestRigPost
  road : Outport

== system Vehicle_Dynamics_Tests_org/Wheel RR/Road Inputs ==
  note: 1) Only subsystems can be added as variant choices at this level
      | 2) Blocks cannot be connected at this level as connectivity is
      | automatically determined at simulation, based on the active variant
  Non-moving road : Delft_Tyre_sm2glib/SimMechanics 2G/Non-moving road  VariantControl=NonMoving  dummy=off
  Test Rig Post : Subsystem  VariantControl=TestRigPost
  road : Outport

== system Vehicle_Dynamics_Tests_org/World/Road ==
  note: 1) Only subsystems can be added as variant choices at this level
      | 2) Blocks cannot be connected at this level as connectivity is
      | automatically determined at simulation, based on the active variant
  Bumpy Road : Subsystem  VariantControl=BumpyRoad
  No Road : Subsystem  VariantControl=NoRoad
  B : PMIOPort  Side=Right

== system Vehicle_Dynamics_Tests_org/Wheel LF/Road Inputs/Test Rig Post ==
  Moving Road : Delft_Tyre_sm2glib/SimMechanics 2G/Moving Road sm2G  response_time=0.05  tyre_id=1
  Step road input 1 : Step  Time=3  After=0.05  SampleTime=0
  road : Outport
  wires:
  Moving Road/1 -> road/1
  Step road input 1/1 -> Moving Road/1

== system Vehicle_Dynamics_Tests_org/Wheel LR/Road Inputs/Test Rig Post ==
  Moving Road : Delft_Tyre_sm2glib/SimMechanics 2G/Moving Road sm2G  response_time=0.05  tyre_id=3
  Step road input : Step  Time=5  After=0.05  SampleTime=0
  road : Outport
  wires:
  Moving Road/1 -> road/1
  Step road input/1 -> Moving Road/1

== system Vehicle_Dynamics_Tests_org/Wheel RF/Road Inputs/Test Rig Post ==
  Moving Road : Delft_Tyre_sm2glib/SimMechanics 2G/Moving Road sm2G  response_time=0.05  tyre_id=2
  Step road input 2 : Step  Time=4  After=0.05  SampleTime=0
  road : Outport
  wires:
  Moving Road/1 -> road/1
  Step road input 2/1 -> Moving Road/1

== system Vehicle_Dynamics_Tests_org/Wheel RR/Road Inputs/Test Rig Post ==
  Moving Road : Delft_Tyre_sm2glib/SimMechanics 2G/Moving Road sm2G  response_time=0.05  tyre_id=4
  Step road input : Step  Time=6  After=0.05  SampleTime=0
  road : Outport
  wires:
  Moving Road/1 -> road/1
  Step road input/1 -> Moving Road/1

== system Vehicle_Dynamics_Tests_org/World/Road/Bumpy Road ==
  Left Road : sm_lib/Body Elements/Solid  InertiaType=Custom  Mass=0  MassUnits=kg  CenterOfMass=[0 0 0]  CenterOfMassUnits=m  MomentsOfInertia=[0 0 0]  MomentsOfInertiaUnits=kg*m^2  ProductsOfInertia=[0 0 0]  ProductsOfInertiaUnits=kg*m^2  DensityBased=on  Density=1000  DensityUnits=kg/(m^3)  DoExposeReferenceFrame=on  SerializedFrames=<Frames/>  GraphicType=FromGeometry  MarkerShape=Sphere  MarkerSize=10  MarkerSizeUnits=m  GraphicVisPropType=SimpleVisualProperties  GraphicDiffuseColor=[0.5 0.5 0.5]  GraphicSpecularColor=[0.5 0.5 0.5 1.0]  GraphicAmbientColor=[0.15 0.15 0.15 1.0]  GraphicEmissiveColor=[0.0 0.0 0.0 1.0]  GraphicShininess=75  GraphicOpacity=1.0  GeometryShape=GeneralExtrusion  RectangleSize=[1 1]  RectangleSizeUnits=m  BrickDimensions=[10 10 0.001]  BrickDimensionUnits=m  CylinderRadius=1  CylinderRadiusUnits=m  CylinderLength=1  CylinderLengthUnits=m  SphereRadius=1  SphereRadiusUnits=m  EllipsoidRadii=[1 1 1]  EllipsoidRadiiUnits=m  ExtrusionCrossSection=Road_Extr_Data_L  ExtrusionCrossSectionUnits=m  ExtrusionLength=0.5  ExtrusionLengthUnits=m  PolygonNumSides=4  PolygonOuterRadius=1  PolygonOuterRadiusUnits=m  ExtGeomFileType=STEP  ExtGeomFileUnits=m  RevolutionCrossSection=[1 1; 1 -1; 2 -1; 2 1]  RevolutionCrossSectionUnits=m  RevolutionExtent=Full  RevolutionAngle=180  RevolutionAngleUnits=deg
  Right Road : sm_lib/Body Elements/Solid  InertiaType=Custom  Mass=0  MassUnits=kg  CenterOfMass=[0 0 0]  CenterOfMassUnits=m  MomentsOfInertia=[0 0 0]  MomentsOfInertiaUnits=kg*m^2  ProductsOfInertia=[0 0 0]  ProductsOfInertiaUnits=kg*m^2  DensityBased=on  Density=1000  DensityUnits=kg/(m^3)  DoExposeReferenceFrame=on  SerializedFrames=<Frames/>  GraphicType=FromGeometry  MarkerShape=Sphere  MarkerSize=10  MarkerSizeUnits=m  GraphicVisPropType=SimpleVisualProperties  GraphicDiffuseColor=[0.5 0.5 0.5]  GraphicSpecularColor=[0.5 0.5 0.5 1.0]  GraphicAmbientColor=[0.15 0.15 0.15 1.0]  GraphicEmissiveColor=[0.0 0.0 0.0 1.0]  GraphicShininess=75  GraphicOpacity=1.0  GeometryShape=GeneralExtrusion  RectangleSize=[1 1]  RectangleSizeUnits=m  BrickDimensions=[10 10 0.001]  BrickDimensionUnits=m  CylinderRadius=1  CylinderRadiusUnits=m  CylinderLength=1  CylinderLengthUnits=m  SphereRadius=1  SphereRadiusUnits=m  EllipsoidRadii=[1 1 1]  EllipsoidRadiiUnits=m  ExtrusionCrossSection=Road_Extr_Data_R  ExtrusionCrossSectionUnits=m  ExtrusionLength=0.5  ExtrusionLengthUnits=m  PolygonNumSides=4  PolygonOuterRadius=1  PolygonOuterRadiusUnits=m  ExtGeomFileType=STEP  ExtGeomFileUnits=m  RevolutionCrossSection=[1 1; 1 -1; 2 -1; 2 1]  RevolutionCrossSectionUnits=m  RevolutionExtent=Full  RevolutionAngle=180  RevolutionAngleUnits=deg
  Transform (Ground) : sm_lib/Frames and Transforms/Rigid Transform  TranslationMethod=StandardAxis  TranslationStandardOffset=TNO_Veh_PARAM.WheelBase/2  TranslationLengthUnit=m  TranslationStandardAxis=+Y  TranslationCartesianOffset=[0 0 0]  TranslationROffset=0  TranslationROffsetUnits=m  TranslationZOffset=0  TranslationZOffsetUnits=m  TranslationThetaOffset=0  TranslationThetaOffsetUnits=deg  RotationMethod=StandardAxis  RotationAngleUnits=deg  RotationStandardAxis=+X  RotationAngle=90  RotationArbitraryAxis=[0 0 1]  FollAlignAxisA=+X  BaseAlignAxisA=+Y  FollAlignAxisB=+Y  BaseAlignAxisB=+Z  RotationSequenceAxes=FollowerAxes  RotationSequence=XYX  RotationSequenceAngles=[0 0 0]  RotationSequenceAnglesUnits=deg  RotationMatrix=[1 0 0; 0 1 0; 0 0 1]
  Transform (Ground)1 : sm_lib/Frames and Transforms/Rigid Transform  TranslationMethod=StandardAxis  TranslationStandardOffset=TNO_Veh_PARAM.WheelBase/2  TranslationLengthUnit=m  TranslationStandardAxis=-Y  TranslationCartesianOffset=[0 0 0]  TranslationROffset=0  TranslationROffsetUnits=m  TranslationZOffset=0  TranslationZOffsetUnits=m  TranslationThetaOffset=0  TranslationThetaOffsetUnits=deg  RotationMethod=StandardAxis  RotationAngleUnits=deg  RotationStandardAxis=+X  RotationAngle=90  RotationArbitraryAxis=[0 0 1]  FollAlignAxisA=+X  BaseAlignAxisA=+Y  FollAlignAxisB=+Y  BaseAlignAxisB=+Z  RotationSequenceAxes=FollowerAxes  RotationSequence=XYX  RotationSequenceAngles=[0 0 0]  RotationSequenceAnglesUnits=deg  RotationMatrix=[1 0 0; 0 1 0; 0 0 1]
  B : PMIOPort  Side=Right
  connections:
  Transform (Ground)1/LConn1 -- Transform (Ground)/LConn1 -- B/RConn1
  Transform (Ground)1/RConn1 -- Right Road/RConn1
  Transform (Ground)/RConn1 -- Left Road/RConn1

== system Vehicle_Dynamics_Tests_org/World/Road/No Road ==
  B : PMIOPort  Side=Right
